simulink model "MOD5_Counter"  (R2020a)
settings: Solver=VariableStepAuto  StartTime=0.0  StopTime=50  RelTol=1e-3
undefined symbols (not defined in the file): sigbuilder_block
settings Model: Creator=DELL  LastModifiedBy=DELL

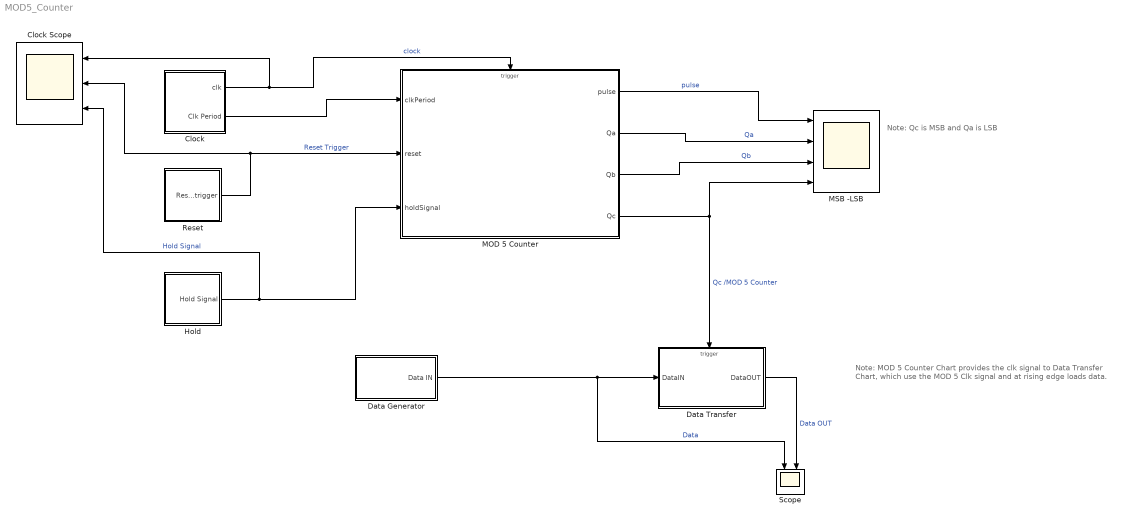
== system MOD5_Counter ==
  note: Note:
      | MOD 5 Counter Chart provides the clk signal to Data Transfer Chart,
      | which use the MOD 5 Clk signal and at rising edge loads data.
  note: Note:
      | Qc is MSB and Qa is LSB
  "Clock " : Subsystem  mask{clkTimePeriod=1}
      mask prompts: clkTimePeriod "Clock Time Period"
      mask DialogControl DescGroupVar Prompt: Clock Details
      mask DialogControl DescTextVar Prompt: Time period of the clock for the counter.
      mask DialogControl ParameterGroupVar Prompt: CLock Paramters
  Clock Scope : Scope  NumInputPorts=3
  Data Generator : Subsystem
  "Data Transfer " : Stateflow chart  TreatAsAtomicUnit=on
  Hold : Subsystem  mask{holdON=22, holdOFF=32}
      mask prompts: holdON "Hold ON Time"; holdOFF "Hold OFF Time"
      mask DialogControl DescGroupVar Prompt: Hold
      mask DialogControl DescTextVar Prompt: The time when to hold the signal from MOD % counter
      mask DialogControl ParameterGroupVar Prompt: Time
  MOD 5 Counter : Stateflow chart  TreatAsAtomicUnit=on
  MSB -LSB : Scope  NumInputPorts=4
  Reset : Subsystem  mask{resetTimeTrigger=12}
      mask prompts: resetTimeTrigger "Reset Trigger Time"
      mask DialogControl DescGroupVar Prompt: Reset Trigger
      mask DialogControl DescTextVar Prompt: Reset the counter to starting.
      mask DialogControl ParameterGroupVar Prompt: Reset Timing Parameter
  Scope : Scope  NumInputPorts=2
  wires:
  MOD 5 Counter/1(pulse) -> MSB -LSB/1  "pulse"
  "Clock "/1(clk) -> Clock Scope/1, MOD 5 Counter/Trigger  "clock"
  "Clock "/2(Clk Period) -> MOD 5 Counter/1(clkPeriod)
  MOD 5 Counter/2(Qa) -> MSB -LSB/2  "Qa"
  MOD 5 Counter/3(Qb) -> MSB -LSB/3  "Qb"
  MOD 5 Counter/4(Qc) -> MSB -LSB/4, "Data Transfer "/Trigger  "Qc /MOD 5 Counter"
  Reset/1(Reset trigger) -> Clock Scope/2, MOD 5 Counter/2(reset)  "Reset Trigger"
  Hold/1(Hold Signal) -> Clock Scope/3, MOD 5 Counter/3(holdSignal)  "Hold Signal"
  "Data Transfer "/1(DataOUT) -> Scope/2  "Data OUT"
  Data Generator/1(Data IN) -> Scope/1, "Data Transfer "/1(DataIN)  "Data"

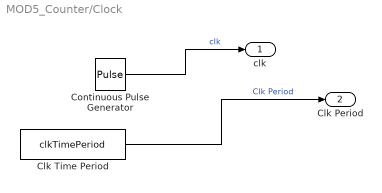
== system MOD5_Counter/Clock  ==
  Clk Time Period : Constant  Value=clkTimePeriod
  Continuous Pulse Generator : DiscretePulseGenerator  PulseType=Time based  Period=clkTimePeriod  PulseWidth=50
  clk : Outport
  Clk Period : Outport  Port=2
  wires:
  Continuous Pulse Generator/1 -> clk/1  "clk"
  Clk Time Period/1 -> Clk Period/1  "Clk Period"

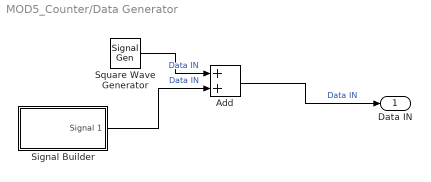
== system MOD5_Counter/Data Generator ==
  Add : Sum
  Signal Builder : Subsystem  Tag=STV Subsys  LoadFcn=sigbuilder_block('load');  StartFcn=sigbuilder_block('start');  StopFcn=sigbuilder_block('stop');  ClipboardFcn=sigbuilder_block('clipboard');  mask(Sigbuilder block){tuvar=[0:10]}
      mask help: Simulink:masks:SigbuilderBlock_MD
      mask init:
      | if ~strcmp(get_param(bdroot(gcbh),'SimulationStatus'),'stopped') tuvar = sigbuilder_block('maskInit'); end
      settings: CopyFcn=sigbuilder_block('copy');  DeleteFcn=sigbuilder_block('delete');  ModelCloseFcn=sigbuilder_block('modelClose');  PreSaveFcn=sigbuilder_block('preSave');  PauseFcn=sigbuilder_block('pause');  ContinueFcn=sigbuilder_block('continue');  NameChangeFcn=sigbuilder_block('namechange');  OpenFcn=sigbuilder_block('open',[393 75 550.8 400.2 ]);  CloseFcn=sigbuilder_block('close');
      mask Display: plot(0, 0, 100, 100,[2, 2, 32, 32, 2], [68, 8, 8, 68, 68],[32, 2], [38, 38], [32, 19, 2],[53, 60, 44], [32, 17, 17, 2],[16, 16, 31, 31]);txt = getActiveGroup(gcbh);text(2, 100, txt,'verticalAlignment', 'top');
  Square Wave Generator : SignalGenerator  WaveForm=square  Units=rad/sec
  Data IN : Outport
  wires:
  Signal Builder/1(Signal 1) -> Add/2  "Data IN"
  Square Wave Generator/1 -> Add/1  "Data IN"
  Add/1 -> Data IN/1  "Data IN"

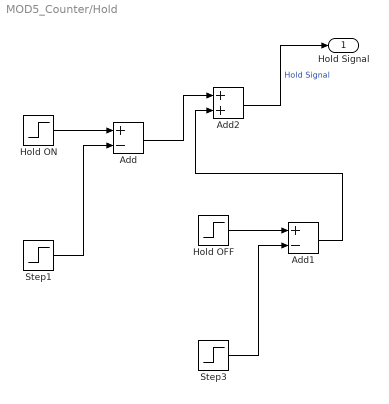
== system MOD5_Counter/Hold ==
  Add : Sum  Inputs=+-
  Add1 : Sum  Inputs=+-
  Add2 : Sum
  Hold OFF : Step  Time=holdOFF  SampleTime=0
  Hold ON : Step  Time=holdON  SampleTime=0
  Step1 : Step  Time=holdON+1  SampleTime=0
  Step3 : Step  Time=holdOFF+1  SampleTime=0
  Hold Signal : Outport
  wires:
  Hold OFF/1 -> Add1/1
  Hold ON/1 -> Add/1
  Step1/1 -> Add/2
  Step3/1 -> Add1/2
  Add1/1 -> Add2/2
  Add/1 -> Add2/1
  Add2/1 -> Hold Signal/1  "Hold Signal"

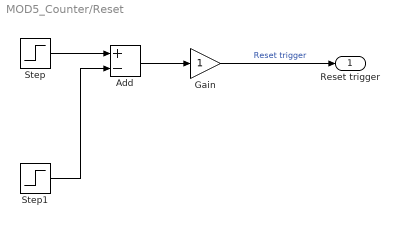
== system MOD5_Counter/Reset ==
  Add : Sum  Inputs=+-
  Gain : Gain
  Step : Step  Time=resetTimeTrigger  SampleTime=0
  Step1 : Step  Time=resetTimeTrigger+1  SampleTime=0
  Reset trigger : Outport
  wires:
  Gain/1 -> Reset trigger/1  "Reset trigger"
  Add/1 -> Gain/1
  Step/1 -> Add/1
  Step1/1 -> Add/2

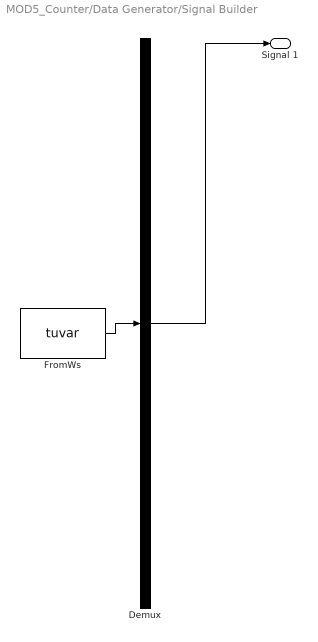
== system MOD5_Counter/Data Generator/Signal Builder ==
  Demux : Demux  Tag=STV Demux  Outputs=1
      settings: DisplayOption=none
  FromWs : FromWorkspace  Tag=STV FromWs  VariableName=tuvar
      SigBuilderData=|
      | common.afterFinalStr = 'Extrapolate'
      | common.sampleTime = 0
      | dataSet.timeRange = [0 50]
      | dataSet.name = 'Group 1'
      | sbobj.Groups.Name = 'Group 1'
      | sbobj.Groups.Signals.Name = 'Signal 1'
      | sbobj.Groups.Signals.XData = [0 4 4 6 6 9.2 12.7 23 32.6 42.4 50]
      | sbobj.Groups.Signals.YData = [0 0 1 1 0 0 2 3 0 0 0]
      | sbobj.Groups.TimeRange = [0 50]
  Signal 1 : Outport  Tag=STV Outport
  wires:
  Demux/1 -> Signal 1/1
  FromWs/1 -> Demux/1

== stateflow chart MOD5_Counter/Data Transfer  ==
  (default) -> (junction 19) : % To carry input
  (junction 19) -> (junction 20) [order 1] : [MOD5CLK]
  (junction 19) -> (junction 21) [order 2]
  (junction 20) -> (junction 22) : {DataOUT = DataIN;}
  (junction 22) -> (junction 21)
  (junction 21) -> (junction 23)
  data: DataIN input; DataOUT output
  events: MOD5CLK input RISING_EDGE_EVENT

== stateflow chart MOD5_Counter/MOD 5 Counter ==
  settings: executeAtInitialization=1
  state CounterON
    HoldSignalLocal = 1;
    (history)
    state State06
      ex:
      Qc = 1;
      Qb = 1;
      Qa = 0;
      pulse =6;
    state State05
      ex:
      Qc = 1;
      Qb = 0;
      Qa = 1;
      pulse =5;
    state State04
      ex:
      Qc = 1;
      Qb = 0;
      Qa = 0;
      pulse =4;
    state State01
      ex:
      Qc = 0;
      Qb = 0;
      Qa = 1;
      pulse =1;
    state State02
      ex:
      Qc = 0;
      Qb = 1;
      Qa = 0;
      pulse =2;
    state State00
      ex:
      Qc = 0;
      Qb = 0;
      Qa = 0;
      pulse =0 ;
    state State03
      ex:
      Qc = 0;
      Qb = 1;
      Qa = 1;
      pulse =3;
    state Reset
      en:
      Qa=0;Qb=0;Qc=0;
      pulse = 0;
    (junction 105) -> (junction 106)
    (junction 106) -> (junction 107)
    (junction 107) -> (junction 108)
    State06 -> (junction 105) [order 1] : [reset == 1]
    State05 -> (junction 106) [order 1] : [reset == 1]
    State04 -> (junction 107) [order 1] : [reset == 1]
    (junction 108) -> (junction 104)
    State04 -> State05 [order 2] : clk
    State05 -> State06 [order 2] : clk
    State03 -> State04 [order 2] : clk
    State06 -> State01 [order 2] : after(clkPeriod/4,sec)
    (default) -> State00
    State02 -> State03 [order 2] : clk
    State01 -> State02 [order 2] : clk
    State00 -> State01 : clk
    State03 -> (junction 103) [order 1] : [reset == 1]
    Reset -> State00 : clk
    State02 -> (junction 101) [order 1] : [reset == 1]
    State01 -> (junction 102) [order 1] : [reset == 1]
    (junction 102) -> Reset
    (junction 101) -> (junction 102)
    (junction 103) -> (junction 101)
    (junction 104) -> (junction 103)
  state Hold
    during:
    HoldSignalLocal = 0;
  (default) -> CounterON
  CounterON -> Hold : [holdSignal == 1 && HoldSignalLocal ==1]
  Hold -> CounterON : [holdSignal == 1 && HoldSignalLocal == 0]
  data: pulse output; clkPeriod input; Qa output; Qb output; Qc output; reset input; HoldSignalLocal local; holdSignal input
  events: clk input RISING_EDGE_EVENT
